simulink model "entri"  (R2022b)
settings: Solver=VariableStepAuto  StartTime=0.0  StopTime=10.0  MaxStep=0.01  RelTol=1e-3
settings Model: Creator=Brigosha_Guest  LastModifiedBy=Brigosha_Guest

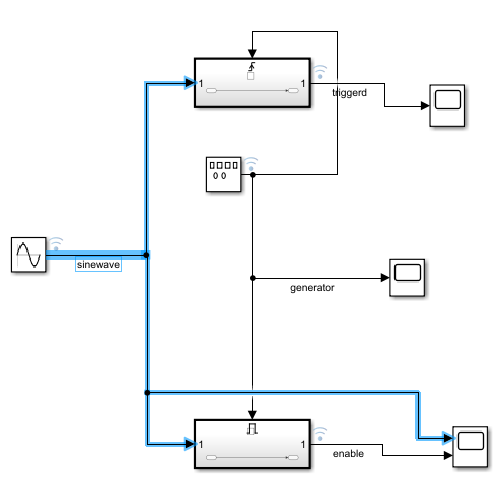
[thumbnail: Simulink's stored preview of the top-level diagram]
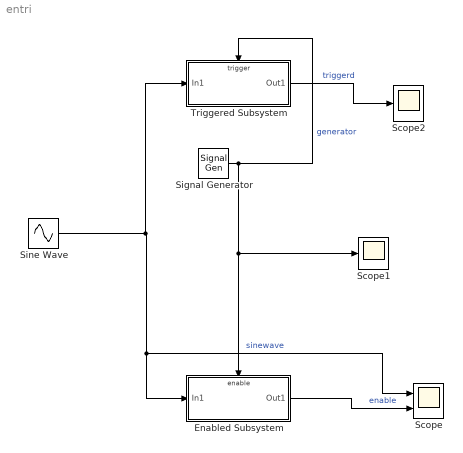
== system entri ==
  Enabled Subsystem : Subsystem  TreatAsAtomicUnit=on
  Scope : Scope  NumInputPorts=2
  Scope1 : Scope
  Scope2 : Scope
  Signal Generator : SignalGenerator  WaveForm=square  Frequency=2.5  Units=rad/sec
  Sine Wave : Sin  SampleTime=0
  Triggered Subsystem : Subsystem  TreatAsAtomicUnit=on
  wires:
  Sine Wave/1 -> Triggered Subsystem/1(In1), Enabled Subsystem/1(In1), Scope/1  "sinewave"
  Enabled Subsystem/1(Out1) -> Scope/2  "enable"
  Signal Generator/1 -> Enabled Subsystem/Enable, Scope1/1, Triggered Subsystem/Trigger  "generator"
  Triggered Subsystem/1(Out1) -> Scope2/1  "triggerd"

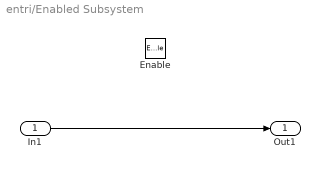
== system entri/Enabled Subsystem ==
  In1 : Inport
  Enable : EnablePort  StatesWhenEnabling=reset
  Out1 : Outport
  wires:
  In1/1 -> Out1/1

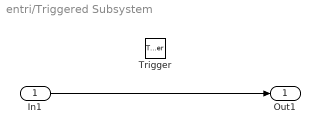
== system entri/Triggered Subsystem ==
  In1 : Inport
  Trigger : TriggerPort  VariantControl=(inherit)  InitialTriggerSignalState=positive
  Out1 : Outport
  wires:
  In1/1 -> Out1/1
